simulink model "PVWIND"  (R2018a)
settings: Solver=FixedStepAuto  StartTime=0.0  StopTime=8  FixedStep=1e-4  RelTol=1e-3  EnableMultiTasking=on
InitFcn:
  | %clear all ;
  | %clc;
  | 
  | %%Wind System%%
  | 
  | %wind speed
  | Z_data=10;
  | Z_hub=85;
  | Z_0=0.03;
  | 
  | %Turbine
  | R_=45;
  | G=100;
  | lambda_opt=7.07;
  | Rho=1.225;
  | J=254;
  | f=0.01;
  | 
  | %RL filter;
  | 
  | fs=10000;
  | fe=50;
  | Ws=2*pi*fe;
  | Pres=3e6;
  | L=0.75e-3;
  | R=0.075;
  | c=38e-3;
  | 
  | %Commande CCR;
  | 
  | Id_=0;
  | Vdc_=1200;
  | %Vq_=0;
  | tr=0.001;
  | kp=3*L/tr;
  | ki=3*R/tr;
  | 
  | %CCM Commande;
  | 
  | p=2;
  | Tr=0.02;
  | Lfs=121e-6;
  | Lfr=57.3e-6;
  | Lm=12.12e-3;
  | m=1;
  | Ls=Lfs+Lm;
  | Lr=Lfr+m*Lm;
  | sigma=1-(m*Lm)^2/(Ls*Lr);
  | Rr=3.82e-3;
  | Rs=2.97e-3;
  | kpr=3*sigma*Lr/Tr;
  | kir=3*Rr/Tr;
  | Qs_ref=0;
  | 
  | %%PV SYSTEM%%
  | 
  | % T_cellule;
  | NOCT=45;
  | 
  | %PV module;
  | ... (+42 lines)
undefined symbols (not defined in the file or in its folder): sigbuilder_block
libraries: simulink x10, powerlib_meascontrol x10
(part 2 of 2)

== matlab function PVWIND/Gm/Irradiation ==
  data: i input; k input; y output; o input; p input
function y = fcn(i,k,o,p)
%Solar irradiation
%k=DNI   o=DHI    p=GHI
n=0;
phi=27.87429;            %latitude
L_st=0;           %standard meridian 
L_loc=-0.29388;          %longitude
c=0;              %daylight savings
theta_m=23;        %tilt angle
phi_m=180;          %solar module azimuth
rho=0.2;            %ground albedo
T_off=1;          %time difference

SVF=0.5*(1+cosd(theta_m));
G_gnd=p*rho*(1-SVF);


 
  n=ceil(i/24);
  C=0.095+0.04*sind(360*(n-100)/365);
  delta=23.45*sind(360*(n-80)/365);  
  B=(n-1)*360/365;
  ET=229.2*(0.000075+0.001868*cosd(B)-0.032077*sind(B)-0.014615*cosd(2*B)-0.04089*sind(2*B));
  %cos(w_)=-tan(phi)+tan(delta);
  G_dif=C*o*SVF;
  
  
      
      UT=(i/24-fix(i/24))*24-T_off;
      t=UT+ET+4*(L_st-L_loc)+c;
      w=15*(t-12);
      D=sind(delta)*sind(phi)+cosd(delta)*cosd(phi)*cosd(w);              %sin(a)
      
      %E=sin(phi)*sin(delta)+cos(phi)*cos(delta)*cos(w);             %cos(theta_z)
      %z=x*E+y;                                                      %GHI
      A=(cosd(phi)*sind(delta)-cosd(delta)*sind(phi)*cosd(w))/cosd(asind(D));     %cos(phi_s')
      
      
if w>0
    
    phi_s=360-acosd(complex(A));
    
else
    
    phi_s=acosd(complex(A));
    
end

      F=cosd(asind(complex(D)))*cosd(phi_s-phi_m)*sind(theta_m)+D*cosd(theta_m);    %cos(gama)
      G_dir=k*F;
      
if G_dir<0
    
     G_dir=-G_dir;
   
end
          
      G=G_dir+G_dif+G_gnd;
    
y = real(G);

== matlab function PVWIND/MPPT2/CI ==
  data: DV input; DP input; d output
function d=PO(DV,DP)
persistent   v ;

if isempty(v)
    v=37.9;
end

if(DP==0)
else
    if(DP>0)
        if(DV>0)
                v=v+0.01;
            else
                v=v-0.01;
           end 
       else
        if(DV>0)
                v=v-0.01;
            else
                v=v+0.01;
        end
    end
end
if(v<25)
    v=25;
end
if(v>45)
    v=45;
end

d=v;
end
